simulink model "onepulserect"  (R2014a)
settings: Solver=ode3  StartTime=0.0  StopTime=0.1  FixedStep=0.0001  RelTol=1e-3
libraries: fl_lib x6, nesl_utility x4, pe_lib x1
settings Model: Creator=Sergey Litvinov  LastModifiedBy=Sergey Litvinov

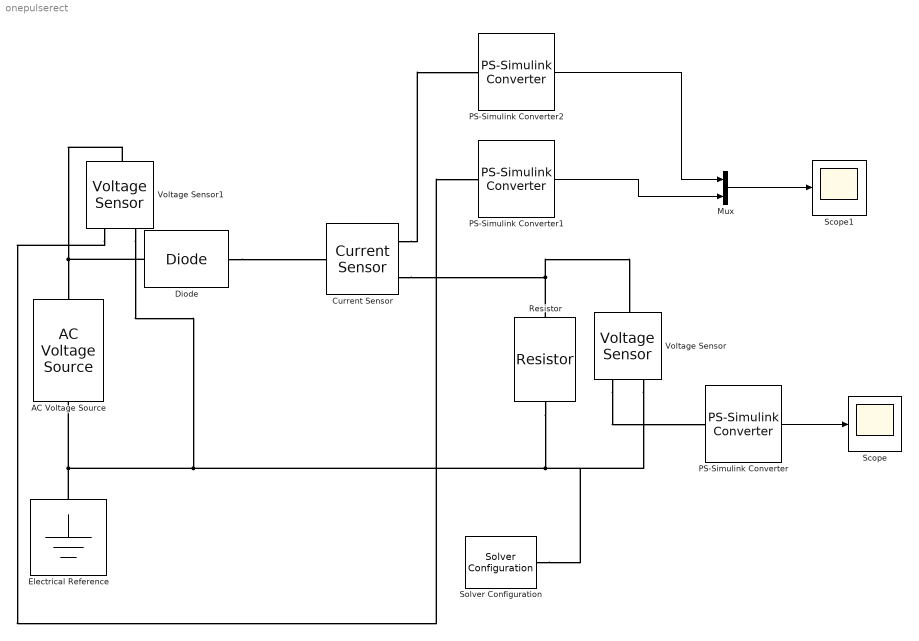
== system onepulserect ==
  AC Voltage Source : fl_lib/Electrical/Electrical Sources/AC Voltage Source  amp=300 V  shift=0 deg  frequency=50 Hz  omega=0 rad/s
  Current Sensor : fl_lib/Electrical/Electrical Sensors/Current Sensor
  Diode : pe_lib/Semiconductors/Fundamental Components/Diode  Vf=0.8 V  Ron=0.001 Ohm  Goff=1e-5 1/Ohm  N_series=1  N_parallel=1  Vf_equiv=0.8 V  Ron_equiv=0.001 Ohm  Goff_equiv=1e-5 1/Ohm
  Electrical Reference : fl_lib/Electrical/Electrical Elements/Electrical Reference
  Mux : Mux  Inputs=2
  PS-Simulink Converter : nesl_utility/PS-Simulink Converter  PhysicalDomain=network_engine_domain  SubClassName=ps_output  LeftPortType=input  RightPortType=output  PseudoPeriodic=off  Frequencies=[]  Unit=1  AffineConversion=off
  PS-Simulink Converter1 : nesl_utility/PS-Simulink Converter  PhysicalDomain=network_engine_domain  SubClassName=ps_output  LeftPortType=input  RightPortType=output  PseudoPeriodic=off  Frequencies=[]  Unit=1  AffineConversion=off
  PS-Simulink Converter2 : nesl_utility/PS-Simulink Converter  PhysicalDomain=network_engine_domain  SubClassName=ps_output  LeftPortType=input  RightPortType=output  PseudoPeriodic=off  Frequencies=[]  Unit=1  AffineConversion=off
  Resistor : fl_lib/Electrical/Electrical Elements/Resistor  R=2 Ohm  i_specify=off  i_priority=High  i=0 A  v_specify=off  v_priority=High  v=0 V
  Scope : Scope
  Scope1 : Scope
  Solver Configuration : nesl_utility/Solver Configuration  PhysicalDomain=network_engine_domain  SubClassName=solver  LeftPortType=input  RightPortType=generic  Accelerate=off  Tones=[]  Harmonics=[]  SimulateNoise=off  Profile=off  UseLocalSampling=off  EnableSwitchedLinearOptims=on  FrequencyDomain=off  UseCCode=off  RelTol=0.001  AbsTol=1e-06  MinStep=1e-09  ToWorkspace=off  DoDC=off  ResidualTolerance=1e-09  UseLocalSolver=off  LocalSolverChoice=NE_BACKWARD_EULER_ADVANCER  LocalSolverSampleTime=0.001  DoFixedCost=off  MaxNonlinIter=3  MaxModeIter=2  LinearAlgebra=Sparse  DelaysMemoryBudget=1024  AutomaticFiltering=on  FilteringTimeConstant=0.001
  Voltage Sensor : fl_lib/Electrical/Electrical Sensors/Voltage Sensor
  Voltage Sensor1 : fl_lib/Electrical/Electrical Sensors/Voltage Sensor
  wires:
  PS-Simulink Converter/1 -> Scope/1
  Mux/1 -> Scope1/1
  PS-Simulink Converter1/1 -> Mux/2
  PS-Simulink Converter2/1 -> Mux/1
  connections:
  Electrical Reference/LConn1 -- Voltage Sensor1/RConn2 -- Solver Configuration/RConn1 -- Voltage Sensor/RConn2 -- Resistor/RConn1 -- AC Voltage Source/RConn1
  Diode/LConn1 -- Voltage Sensor1/LConn1 -- AC Voltage Source/LConn1
  Resistor/LConn1 -- Voltage Sensor/LConn1 -- Current Sensor/RConn2
  Voltage Sensor/RConn1 -- PS-Simulink Converter/LConn1
  Voltage Sensor1/RConn1 -- PS-Simulink Converter1/LConn1
  Diode/RConn1 -- Current Sensor/LConn1
  Current Sensor/RConn1 -- PS-Simulink Converter2/LConn1
